simulink model "TekmaModel"  (R2020b)
settings: Solver=VariableStepAuto  StartTime=0.0  StopTime=120  RelTol=1e-3
undefined symbols (not defined in the file or in its folder): f0, J, k1, k2, k3, lm, psi_1, psi_2
settings Model: Creator=Acer  LastModifiedBy=Acer

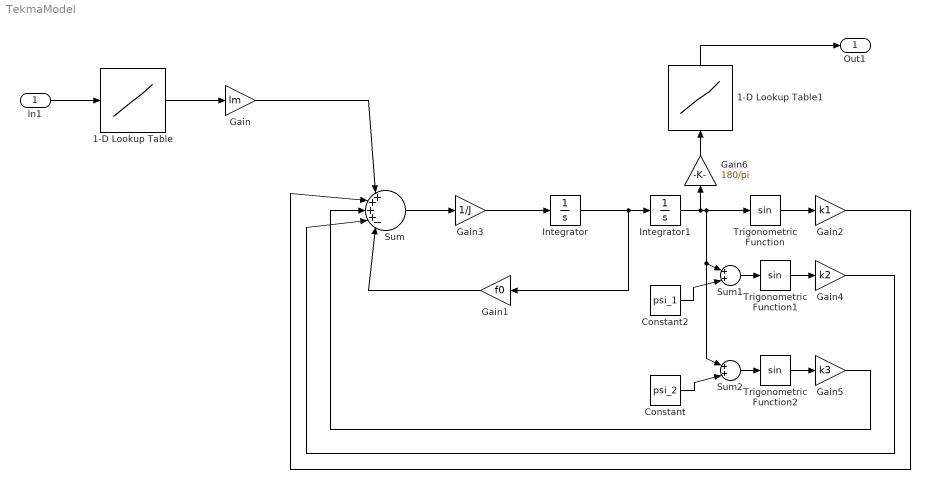
== system TekmaModel ==
  In1 : Inport
  1-D Lookup Table : Lookup_n-D  NumberOfTableDimensions=1  BreakpointsForDimension1=[0,4.6, 4.7, 5, 5.5, 6, 7, 7.5, 8, 8.5, 10]  Table=[0,0,0.10984,0.21163,0.38639,0.54977,0.83,0.9284,0.9284, 0.9284,0.9284]  InternalRulePriority=Speed  RndMeth=Simplest  InputSameDT=on
  1-D Lookup Table1 : Lookup_n-D  NumberOfTableDimensions=1  BreakpointsForDimension1=[14, 90, 177]  Table=[6, 3.52, 0.83]  SampleTime=0.1  InternalRulePriority=Speed  RndMeth=Simplest  InputSameDT=on
  Constant : Constant  Value=psi_2
  Constant2 : Constant  Value=psi_1
  Gain : Gain  Gain=lm
  Gain1 : Gain  Gain=f0
  Gain2 : Gain  Gain=k1
  Gain3 : Gain  Gain=1/J
  Gain4 : Gain  Gain=k2
  Gain5 : Gain  Gain=k3
  Gain6 : Gain  Gain=180/pi
  Integrator : Integrator
  Integrator1 : Integrator
  Sum : Sum  Inputs=|++++-|
  Sum1 : Sum  Inputs=|++|
  Sum2 : Sum  Inputs=|++|
  Trigonometric Function : Trigonometry
  Trigonometric Function1 : Trigonometry
  Trigonometric Function2 : Trigonometry
  Out1 : Outport
  wires:
  Gain4/1 -> Sum/4
  Trigonometric Function/1 -> Gain2/1
  Trigonometric Function1/1 -> Gain4/1
  Sum2/1 -> Trigonometric Function2/1
  Integrator/1 -> Integrator1/1, Gain1/1
  Constant/1 -> Sum2/2
  Gain/1 -> Sum/1
  Constant2/1 -> Sum1/2
  Gain3/1 -> Integrator/1
  Gain5/1 -> Sum/3
  1-D Lookup Table/1 -> Gain/1
  Gain1/1 -> Sum/5
  Gain2/1 -> Sum/2
  Sum1/1 -> Trigonometric Function1/1
  In1/1 -> 1-D Lookup Table/1
  Trigonometric Function2/1 -> Gain5/1
  Sum/1 -> Gain3/1
  1-D Lookup Table1/1 -> Out1/1
  Integrator1/1 -> Trigonometric Function/1, Sum2/1, Sum1/1, Gain6/1
  Gain6/1 -> 1-D Lookup Table1/1
